simulink model "dom_schem"  (R2018a)
settings: Solver=VariableStepAuto  StartTime=0.0  StopTime=9000.0  RelTol=1e-3
values from neighbouring files (symbols this model uses):
  c_p = 1000    [dom_script.m]
  C_vp = c_p*ro_p*V_pp    (= 43200)    [dom_script.m]
  C_vw = c_p*ro_p*V_gp    (= 129600)    [dom_script.m]
  f_pn = 1    [dom_script.m]
  ro_p = 1.2    [dom_script.m]
  T_p_0 = 18    [dom_script.m]
  T_wew_0 = 21    [dom_script.m]
  T_zewn = -1    [dom_script.m]
  T_zn = 24    [dom_script.m]
undefined symbols (not defined in the file or in its folder): K_1, K_p, K_w
settings Model: Creator=johnb  LastModifiedBy=john

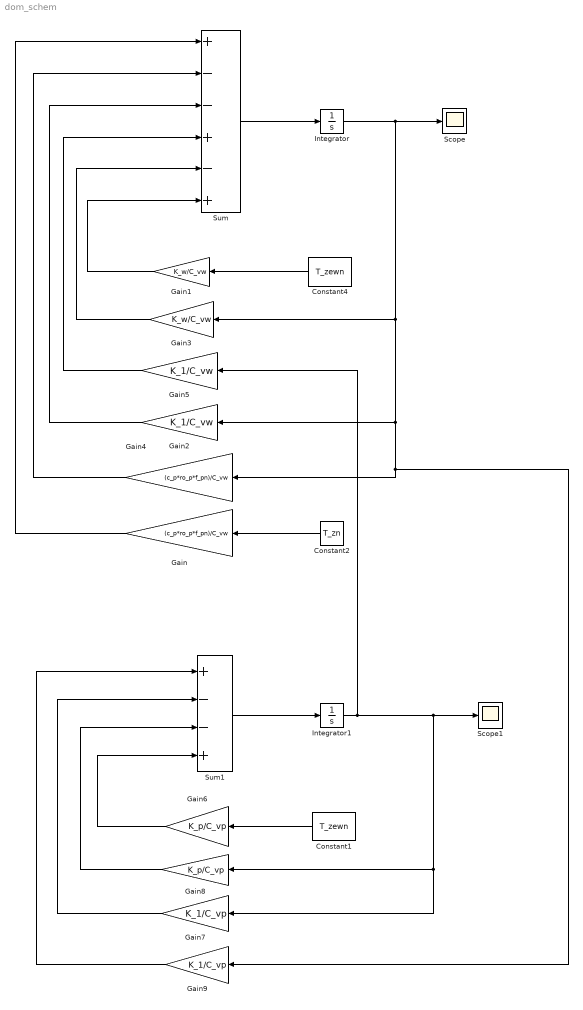
== system dom_schem ==
  Constant1 : Constant  Value=T_zewn
  Constant2 : Constant  Value=T_zn
  Constant4 : Constant  Value=T_zewn
  Gain : Gain  Gain=(c_p*ro_p*f_pn)/C_vw
  Gain1 : Gain  Gain=K_w/C_vw
  Gain2 : Gain  Gain=K_1/C_vw
  Gain3 : Gain  Gain=K_w/C_vw
  Gain4 : Gain  Gain=(c_p*ro_p*f_pn)/C_vw
  Gain5 : Gain  Gain=K_1/C_vw
  Gain6 : Gain  Gain=K_p/C_vp
  Gain7 : Gain  Gain=K_1/C_vp
  Gain8 : Gain  Gain=K_p/C_vp
  Gain9 : Gain  Gain=K_1/C_vp
  Integrator : Integrator  InitialCondition=T_wew_0
  Integrator1 : Integrator  InitialCondition=T_p_0
  Scope : Scope
  Scope1 : Scope
  Sum : Sum  Inputs=+--+-+
  Sum1 : Sum  Inputs=+--+
  wires:
  Sum/1 -> Integrator/1
  Constant2/1 -> Gain/1
  Gain/1 -> Sum/1
  Integrator/1 -> Gain3/1, Gain2/1, Gain9/1, Gain4/1, Scope/1
  Gain4/1 -> Sum/2
  Gain2/1 -> Sum/3
  Integrator1/1 -> Gain7/1, Gain8/1, Scope1/1, Gain5/1
  Gain5/1 -> Sum/4
  Gain3/1 -> Sum/5
  Gain1/1 -> Sum/6
  Constant4/1 -> Gain1/1
  Sum1/1 -> Integrator1/1
  Gain9/1 -> Sum1/1
  Gain7/1 -> Sum1/2
  Gain8/1 -> Sum1/3
  Gain6/1 -> Sum1/4
  Constant1/1 -> Gain6/1
